simulink model "Aerosonde"  (R2025b)
settings: Solver=VariableStepAuto  StartTime=0.0  StopTime=100  RelTol=1e-3
values from neighbouring files (symbols this model uses):
  b = 2.8956    [init_params.m]    (also in init_params.mat)
  c = 0.18994    [init_params.m]    (also in init_params.mat)
  Cprop = 1.0    (= 1)    [init_params.m]    (also in init_params.mat)
  del_a = 0    [StatesAndInputs.m]
  del_e = 2*(pi/180)    (= 0.0349065850399)    [StatesAndInputs.m]
  del_r = 0    [StatesAndInputs.m]
  ForceCoefficients = [0.28 3.45 0 -0.36 0.03 0.3 0 0 0.0437 0 -0.98 0 ... (15 elements, 15x1)]    [init_params.mat]
  g = 9.80665    [init_params.m]    (also in init_params.mat)
  Ixx = 0.8244    [init_params.m]    (also in init_params.mat)
  Ixz = 0.1204    [init_params.m]    (also in init_params.mat)
  Iyy = 1.135    [init_params.m]    (also in init_params.mat)
  Izz = 1.759    [init_params.m]    (also in init_params.mat)
  k_motor = 80    [init_params.m]    (also in init_params.mat)
  k_omega = 0    [init_params.m]    (also in init_params.mat)
  k_Tp = 0    [init_params.m]    (also in init_params.mat)
  m = 13.5    [init_params.m]    (also in init_params.mat)
  MomentCoefficients = [0 -0.12 -0.26 0.14 0.08 0.105 -0.02338 -0.38 -3.6 -0.5 0 0.25 ... (16 elements, 16x1)]    [init_params.mat]
  p = 0    [StatesAndInputs.m]
  phi = 0    [StatesAndInputs.m]
  psi = 0    [StatesAndInputs.m]
  q = 0    [StatesAndInputs.m]
  r = 0    [StatesAndInputs.m]
  rho = 1.2682    [init_params.m]    (also in init_params.mat)
  S = 0.55    [init_params.m]    (also in init_params.mat)
  S_prop = 0.2027    [init_params.m]    (also in init_params.mat)
  theta = 3*(pi/180)    (= 0.0523598775598)    [StatesAndInputs.m]
  v = 0    [StatesAndInputs.m]
  w = 0    [StatesAndInputs.m]
  x = 0    [StatesAndInputs.m]
  y = 0    [StatesAndInputs.m]
  z = -50    [StatesAndInputs.m]
libraries: matrix_library x2, slpidlib x1
settings Model: Creator=deepa  LastModifiedBy=deepa
settings DataIOCC: ExternalInput=getinputstruct(op1)  InitialState=getstatestruct(op1)

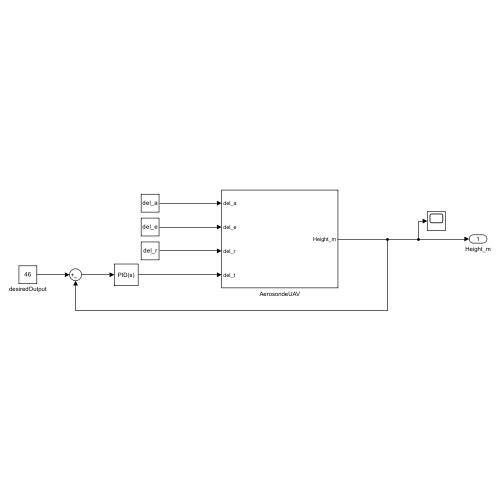
[thumbnail: Simulink's stored preview of the top-level diagram]
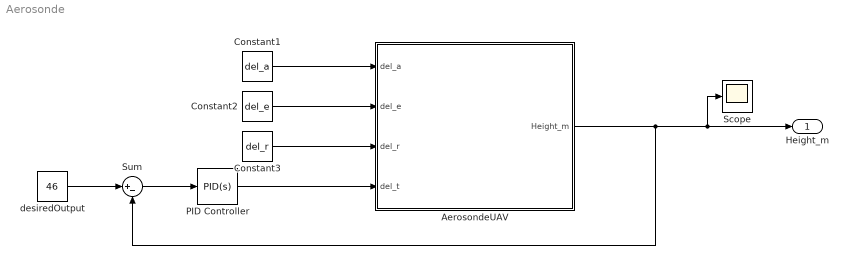
== system Aerosonde ==
  AerosondeUAV : Subsystem
  Constant1 : Constant  Value=del_a
  Constant2 : Constant  Value=del_e
  Constant3 : Constant  Value=del_r
  PID Controller : slpidlib/PID Controller  Controller=PID  Form=Parallel  TimeDomain=Continuous-time  UseExternalTs=off  SampleTime=-1  IntegratorMethod=Forward Euler  FilterMethod=Forward Euler  ControllerParametersSource=internal  P=1  I=1  UseKiTs=off  D=0  UseExternalDerivativeSource=off  N=100  UseFilter=on  TunerSelectOption=Transfer Function Based (PID Tuner App)  InitialConditionSource=internal  InitialConditionForIntegrator=0  InitialConditionForFilter=0  DifferentiatorICPrevScaledInput=0  ExternalReset=none  TrackingMode=off  Kt=1  LimitOutput=off  SatLimitsSource=internal  UpperSaturationLimit=inf  LowerSaturationLimit=-inf  LinearizeAsGain=on  AntiWindupMode=none  Kb=1  LimitIntegrator=off  UpperIntegratorSaturationLimit=inf  LowerIntegratorSaturationLimit=-inf  POutMin=[]  POutMax=[]  IOutMin=[]  IOutMax=[]  DOutMin=[]  DOutMax=[]  NOutMin=[]  NOutMax=[]  SumOutMin=[]  SumOutMax=[]  SaturationOutMin=[]  SaturationOutMax=[]  PParamMin=[]  PParamMax=[]  IParamMin=[]  IParamMax=[]  DParamMin=[]  DParamMax=[]  NParamMin=[]  NParamMax=[]  KbParamMin=[]  KbParamMax=[]  KtParamMin=[]  KtParamMax=[]  KbOutMin=[]  KbOutMax=[]  KtOutMin=[]  KtOutMax=[]  IntegratorOutMin=[]  IntegratorOutMax=[]  FilterOutMin=[]  FilterOutMax=[]  SumI1OutMin=[]  SumI1OutMax=[]  SumI2OutMin=[]  SumI2OutMax=[]  SumI3OutMin=[]  SumI3OutMax=[]  SumI4OutMin=[]  SumI4OutMax=[]  SumDOutMin=[]  SumDOutMax=[]  DifferentiatorOutMin=[]  DifferentiatorOutMax=[]  FilterDiffOutCoefMin=[]  FilterDiffOutCoefMax=[]  ReciprocalOutMin=[]  ReciprocalOutMax=[]  SumDenOutMin=[]  SumDenOutMax=[]  SumNumOutMin=[]  SumNumOutMax=[]  DivideOutMin=[]  DivideOutMax=[]  UdiffTsProdOutMin=[]  UdiffTsProdOutMax=[]  NTsProdOutMin=[]  NTsProdOutMax=[]  UintegralTsProdOutMin=[]  UintegralTsProdOutMax=[]  UngainTsProdOutMin=[]  UngainTsProdOutMax=[]  ClampingZeroOutDataTypeStr=Inherit: Inherit via back propagation  ClampingZeroOutMin=[]  ClampingZeroOutMax=[]  FilterDenConstantOutDataTypeStr=Inherit: Inherit via back propagation  FilterDenConstantOutMin=[]  FilterDenConstantOutMax=[]  PCopyOutDataTypeStr=Inherit: Inherit via back propagation  PCopyOutMin=[]  PCopyOutMax=[]  NCopyOutDataTypeStr=Inherit: Inherit via back propagation  NCopyOutMin=[]  NCopyOutMax=[]  IntegratorContinuousStateAttributes=''  IntegratorStateMustResolveToSignalObject=off  IntegratorRTWStateStorageClass=Auto  FilterContinuousStateAttributes=''  FilterStateMustResolveToSignalObject=off  FilterRTWStateStorageClass=Auto  ParallelPVariant=InternalParameters  IdealPVariant=Disabled  IVariant=InternalParameters  DVariant=InternalParameters  IntegratorVariant=Continuous  SatVariant=Disabled  AWVariant=Passthrough  PCopyVariant=Disabled  TRVariant=Disabled  FdbkBlocksVariant=Forward  IdealPFdbkVariant=Disabled  SatFdbkVariant=Disabled  DerivativeFilterVariant=ContFilter  NVariant=InternalParameters  NCopyVariant=Disabled  FilterICVariant=InternalICsFilter  IntegratorICVariant=InternalICs  ExternalResetVariant=Disabled  TRSumVariant=Passthrough  SumFdbkVariant=Disabled  SumVariant=Sum_PID  TsampFilterVariant=InternalTs  TsampNgainVariant=Passthrough  TsampIntegralVariant=Disabled_SignalSpec  ExternalSaturationOutDataTypeStr=Inherit: Same as second input  DerivativeSourceVariant=ErrorSignal  PreIntVariant=InternalPreInt
  Scope : Scope
      settings: ActiveDisplayYMinimum=-50.13744  ActiveDisplayYMaximum=-48.97284
  Sum : Sum  Inputs=|+-
  desiredOutput : Constant  Value=46
  Height_m : Outport
  wires:
  AerosondeUAV/1(Height_m) -> Sum/2, Scope/1, Height_m/1
  desiredOutput/1 -> Sum/1
  Constant1/1 -> AerosondeUAV/1(del_a)
  Constant2/1 -> AerosondeUAV/2(del_e)
  Constant3/1 -> AerosondeUAV/3(del_r)
  Sum/1 -> PID Controller/1
  PID Controller/1 -> AerosondeUAV/4(del_t)

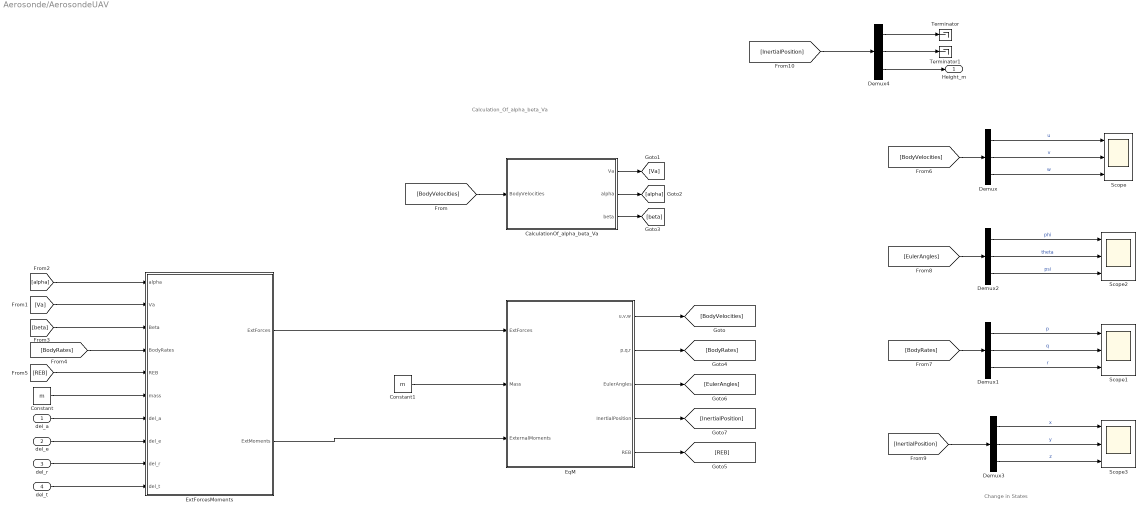
== system Aerosonde/AerosondeUAV ==
  note: Calculation_Of_alpha_beta_Va
  note: Change in States
  del_a : Inport
  del_e : Inport  Port=2
  del_r : Inport  Port=3
  del_t : Inport  Port=4
  CalculationOf_alpha_beta_Va : Subsystem
  Constant : Constant  Value=m
  Constant1 : Constant  Value=m
  Demux{,1..4} (5 alike) : Demux  Outputs=3
  EqM : Subsystem
  ExtForcesMoments : Subsystem
  Scope{,1..3} (4 alike) : Scope  NumInputPorts=3
      Scope settings: ActiveDisplayYMinimum=-68.28294  ActiveDisplayYMaximum=365.82044
      Scope1 settings: ActiveDisplayYMinimum=-3981.32854  ActiveDisplayYMaximum=442.36984
      Scope2 settings: ActiveDisplayYMinimum=-30055.42202  ActiveDisplayYMaximum=3339.54951  DataLoggingVariableName=ScopeData2
      Scope3 settings: ActiveDisplayYMinimum=-56.3817  ActiveDisplayYMaximum=7.22544  DataLoggingVariableName=ScopeData3
  Terminator : Terminator
  Terminator1 : Terminator
  Height_m : Outport
  wires:
  Constant/1 -> ExtForcesMoments/6(mass)
  EqM/3(EulerAngles) -> [EulerAngles]
  [beta] -> ExtForcesMoments/3(Beta)
  [InertialPosition] -> Demux3/1
  del_a/1 -> ExtForcesMoments/7(del_a)
  Demux4/2 -> Terminator1/1
  [REB] -> ExtForcesMoments/5(REB)
  EqM/2(p,q,r) -> [BodyRates]
  [Va] -> ExtForcesMoments/2(Va)
  Demux2/1 -> Scope2/1  "phi"
  Demux/2 -> Scope/2  "v"
  Demux3/2 -> Scope3/2  "y"
  Demux3/1 -> Scope3/1  "x"
  del_r/1 -> ExtForcesMoments/9(del_r)
  [BodyRates] -> ExtForcesMoments/4(BodyRates)
  [BodyRates] -> Demux1/1
  Constant1/1 -> EqM/2(Mass)
  CalculationOf_alpha_beta_Va/3(beta) -> [beta]
  [BodyVelocities] -> CalculationOf_alpha_beta_Va/1(BodyVelocities)
  [alpha] -> ExtForcesMoments/1(alpha)
  Demux3/3 -> Scope3/3  "z"
  Demux1/2 -> Scope1/2  "q"
  Demux/3 -> Scope/3  "w"
  Demux2/3 -> Scope2/3  "psi"
  Demux1/1 -> Scope1/1  "p"
  Demux/1 -> Scope/1  "u"
  EqM/4(InertialPosition) -> [InertialPosition]
  ExtForcesMoments/1(ExtForces) -> EqM/1(ExtForces)
  Demux2/2 -> Scope2/2  "theta"
  del_e/1 -> ExtForcesMoments/8(del_e)
  EqM/5(REB) -> [REB]
  EqM/1(u,v,w) -> [BodyVelocities]
  CalculationOf_alpha_beta_Va/1(Va) -> [Va]
  ExtForcesMoments/2(ExtMoments) -> EqM/3(ExternalMoments)
  [BodyVelocities] -> Demux/1
  CalculationOf_alpha_beta_Va/2(alpha) -> [alpha]
  [EulerAngles] -> Demux2/1
  Demux1/3 -> Scope1/3  "r"
  [InertialPosition] -> Demux4/1
  Demux4/1 -> Terminator/1
  Demux4/3 -> Height_m/1
  del_t/1 -> ExtForcesMoments/10(del_t)

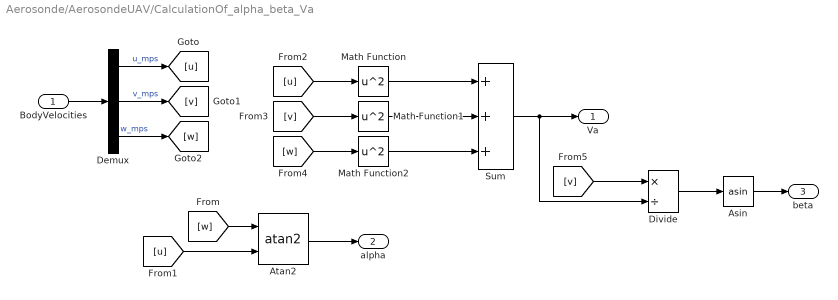
== system Aerosonde/AerosondeUAV/CalculationOf_alpha_beta_Va ==
  BodyVelocities : Inport
  Asin : Trigonometry  Operator=asin
  Atan2 : Trigonometry  Operator=atan2
  Demux : Demux  Outputs=3
  Divide : Product  Inputs=*/
  Math Function : Math  Operator=square
  Math Function1 : Math  Operator=square
  Math Function2 : Math  Operator=square
  Sum : Sum  Inputs=+++
  Va : Outport
  alpha : Outport  Port=2
  beta : Outport  Port=3
  wires:
  BodyVelocities/1 -> Demux/1
  Demux/1 -> [u]  "u_mps"
  Demux/2 -> [v]  "v_mps"
  Demux/3 -> [w]  "w_mps"
  [w] -> Atan2/1
  [u] -> Atan2/2
  Atan2/1 -> alpha/1
  [u] -> Math Function/1
  [v] -> Math Function1/1
  [w] -> Math Function2/1
  Math Function/1 -> Sum/1
  Math Function1/1 -> Sum/2
  Math Function2/1 -> Sum/3
  Sum/1 -> Divide/2, Va/1
  [v] -> Divide/1
  Divide/1 -> Asin/1
  Asin/1 -> beta/1

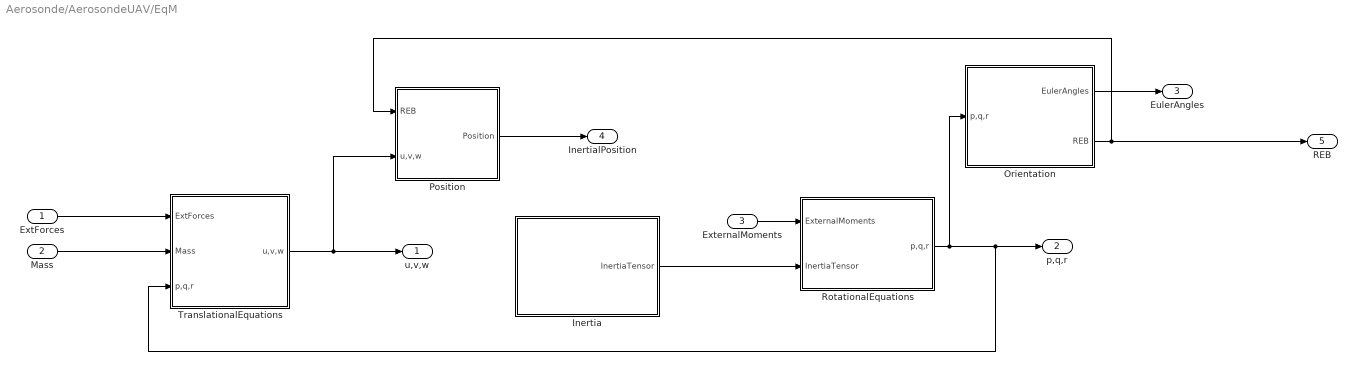
== system Aerosonde/AerosondeUAV/EqM ==
  ExtForces : Inport
  Mass : Inport  Port=2
  ExternalMoments : Inport  Port=3
  Inertia : Subsystem
  Orientation : Subsystem
  Position : Subsystem
  RotationalEquations : Subsystem
  TranslationalEquations : Subsystem
  u,v,w : Outport
  p,q,r : Outport  Port=2
  EulerAngles : Outport  Port=3
  InertialPosition : Outport  Port=4
  REB : Outport  Port=5
  wires:
  Orientation/2(REB) -> Position/1(REB), REB/1
  RotationalEquations/1(p,q,r) -> Orientation/1(p,q,r), p,q,r/1, TranslationalEquations/3(p,q,r)
  ExtForces/1 -> TranslationalEquations/1(ExtForces)
  Mass/1 -> TranslationalEquations/2(Mass)
  TranslationalEquations/1(u,v,w) -> u,v,w/1, Position/2(u,v,w)
  Orientation/1(EulerAngles) -> EulerAngles/1
  ExternalMoments/1 -> RotationalEquations/1(ExternalMoments)
  Inertia/1(InertiaTensor) -> RotationalEquations/2(InertiaTensor)
  Position/1(Position) -> InertialPosition/1

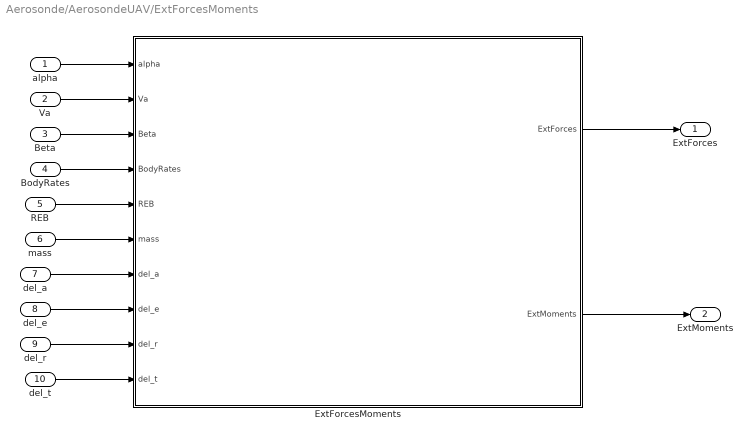
== system Aerosonde/AerosondeUAV/ExtForcesMoments ==
  alpha : Inport
  Va : Inport  Port=2
  Beta : Inport  Port=3
  BodyRates : Inport  Port=4
  REB : Inport  Port=5
  mass : Inport  Port=6
  del_a : Inport  Port=7
  del_e : Inport  Port=8
  del_r : Inport  Port=9
  del_t : Inport  Port=10
  ExtForcesMoments : Subsystem
  ExtForces : Outport
  ExtMoments : Outport  Port=2
  wires:
  alpha/1 -> ExtForcesMoments/1(alpha)
  Va/1 -> ExtForcesMoments/2(Va)
  Beta/1 -> ExtForcesMoments/3(Beta)
  BodyRates/1 -> ExtForcesMoments/4(BodyRates)
  REB/1 -> ExtForcesMoments/5(REB)
  mass/1 -> ExtForcesMoments/6(mass)
  del_a/1 -> ExtForcesMoments/7(del_a)
  del_e/1 -> ExtForcesMoments/8(del_e)
  del_r/1 -> ExtForcesMoments/9(del_r)
  del_t/1 -> ExtForcesMoments/10(del_t)
  ExtForcesMoments/1(ExtForces) -> ExtForces/1
  ExtForcesMoments/2(ExtMoments) -> ExtMoments/1

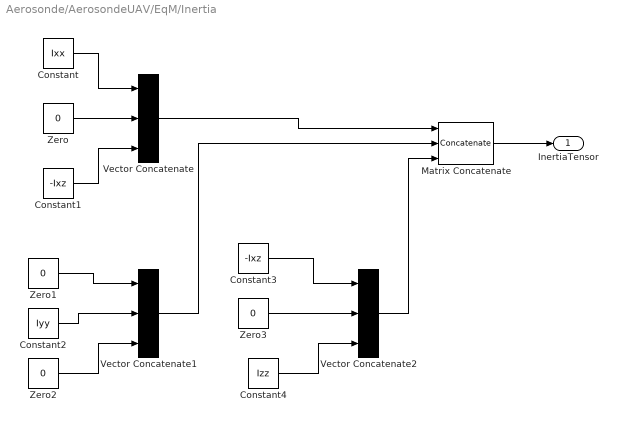
== system Aerosonde/AerosondeUAV/EqM/Inertia ==
  Constant : Constant  Value=Ixx
  Constant1 : Constant  Value=-Ixz
  Constant2 : Constant  Value=Iyy
  Constant3 : Constant  Value=-Ixz
  Constant4 : Constant  Value=Izz
  Matrix Concatenate : Concatenate  NumInputs=3  Mode=Multidimensional array  ConcatenateDimension=2
  Vector Concatenate : Concatenate  NumInputs=3  Mode=Multidimensional array
  Vector Concatenate1 : Concatenate  NumInputs=3  Mode=Multidimensional array
  Vector Concatenate2 : Concatenate  NumInputs=3  Mode=Multidimensional array
  Zero{,1..3} (4 alike) : Constant  Value=0  OutDataTypeStr=Inherit: Inherit via back propagation
  InertiaTensor : Outport
  wires:
  Zero2/1 -> Vector Concatenate1/3
  Constant3/1 -> Vector Concatenate2/1
  Constant2/1 -> Vector Concatenate1/2
  Zero/1 -> Vector Concatenate/2
  Constant1/1 -> Vector Concatenate/3
  Constant/1 -> Vector Concatenate/1
  Zero1/1 -> Vector Concatenate1/1
  Zero3/1 -> Vector Concatenate2/2
  Constant4/1 -> Vector Concatenate2/3
  Vector Concatenate/1 -> Matrix Concatenate/1
  Vector Concatenate1/1 -> Matrix Concatenate/2
  Vector Concatenate2/1 -> Matrix Concatenate/3
  Matrix Concatenate/1 -> InertiaTensor/1

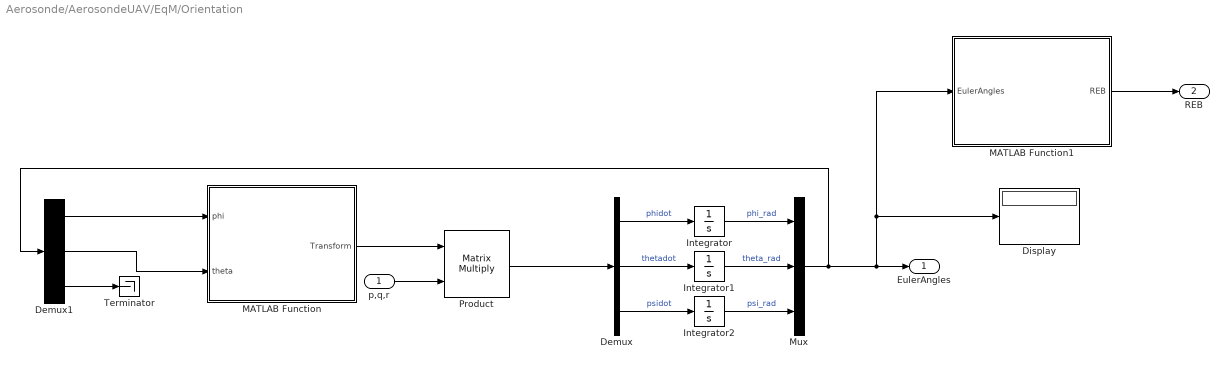
== system Aerosonde/AerosondeUAV/EqM/Orientation ==
  p,q,r : Inport
  Demux : Demux  Outputs=3
  Demux1 : Demux  Outputs=3
  Display : Display
  Integrator : Integrator  InitialCondition=phi  ContinuousStateAttributes='phi_rad'
  Integrator1 : Integrator  InitialCondition=theta  ContinuousStateAttributes='theta_rad'
  Integrator2 : Integrator  InitialCondition=psi  ContinuousStateAttributes='psi_rad'
  MATLAB Function : MATLAB Function  TreatAsAtomicUnit=on
  MATLAB Function1 : MATLAB Function  TreatAsAtomicUnit=on
  Mux : Mux  Inputs=3
  Product : Product  Multiplication=Matrix(*)
  Terminator : Terminator
  EulerAngles : Outport
  REB : Outport  Port=2
  wires:
  MATLAB Function/1(Transform) -> Product/1
  p,q,r/1 -> Product/2
  Product/1 -> Demux/1
  Demux/1 -> Integrator/1  "phidot"
  Demux/2 -> Integrator1/1  "thetadot"
  Demux/3 -> Integrator2/1  "psidot"
  Integrator/1 -> Mux/1  "phi_rad"
  Integrator1/1 -> Mux/2  "theta_rad"
  Integrator2/1 -> Mux/3  "psi_rad"
  Mux/1 -> Demux1/1, MATLAB Function1/1(EulerAngles), Display/1, EulerAngles/1
  MATLAB Function1/1(REB) -> REB/1
  Demux1/1 -> MATLAB Function/1(phi)
  Demux1/2 -> MATLAB Function/2(theta)
  Demux1/3 -> Terminator/1

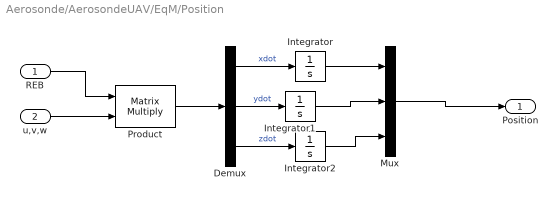
== system Aerosonde/AerosondeUAV/EqM/Position ==
  REB : Inport
  u,v,w : Inport  Port=2
  Demux : Demux  Outputs=3
  Integrator : Integrator  InitialCondition=x  ContinuousStateAttributes='x_m'
  Integrator1 : Integrator  InitialCondition=y  ContinuousStateAttributes='y_m'
  Integrator2 : Integrator  InitialCondition=z  ContinuousStateAttributes='z_m'
  Mux : Mux  Inputs=3
  Product : Product  Multiplication=Matrix(*)
  Position : Outport
  wires:
  REB/1 -> Product/1
  u,v,w/1 -> Product/2
  Product/1 -> Demux/1
  Demux/1 -> Integrator/1  "xdot"
  Demux/2 -> Integrator1/1  "ydot"
  Demux/3 -> Integrator2/1  "zdot"
  Integrator/1 -> Mux/1
  Integrator1/1 -> Mux/2
  Integrator2/1 -> Mux/3
  Mux/1 -> Position/1

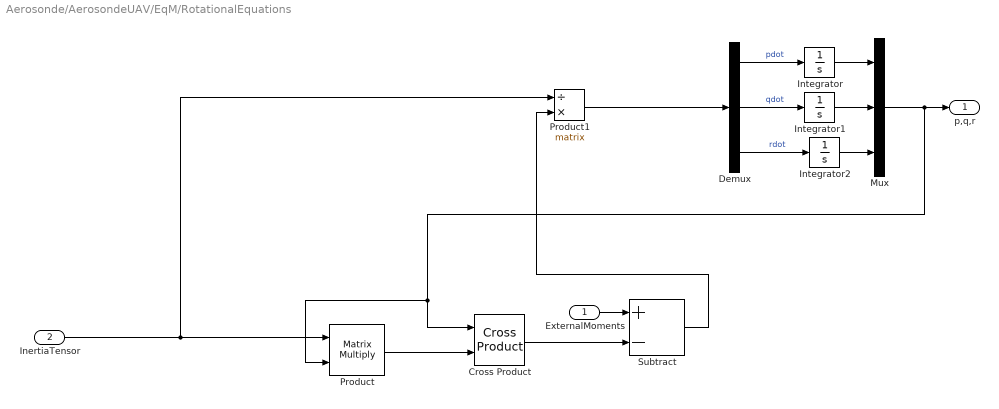
== system Aerosonde/AerosondeUAV/EqM/RotationalEquations ==
  ExternalMoments : Inport
  InertiaTensor : Inport  Port=2
  Cross Product : matrix_library/Cross Product
  Demux : Demux  Outputs=3
  Integrator : Integrator  InitialCondition=p  ContinuousStateAttributes='p_radps'
  Integrator1 : Integrator  InitialCondition=q  ContinuousStateAttributes='q_radps'
  Integrator2 : Integrator  InitialCondition=r  ContinuousStateAttributes='r_radps'
  Mux : Mux  Inputs=3
  Product : Product  Multiplication=Matrix(*)
  Product1 : Product  Inputs=/*  Multiplication=Matrix(*)
  Subtract : Sum  Inputs=+-
  p,q,r : Outport
  wires:
  Mux/1 -> Cross Product/1, Product/2, p,q,r/1
  InertiaTensor/1 -> Product1/1, Product/1
  ExternalMoments/1 -> Subtract/1
  Demux/1 -> Integrator/1  "pdot"
  Demux/2 -> Integrator1/1  "qdot"
  Demux/3 -> Integrator2/1  "rdot"
  Integrator2/1 -> Mux/3
  Integrator1/1 -> Mux/2
  Integrator/1 -> Mux/1
  Cross Product/1 -> Subtract/2
  Product/1 -> Cross Product/2
  Subtract/1 -> Product1/2
  Product1/1 -> Demux/1

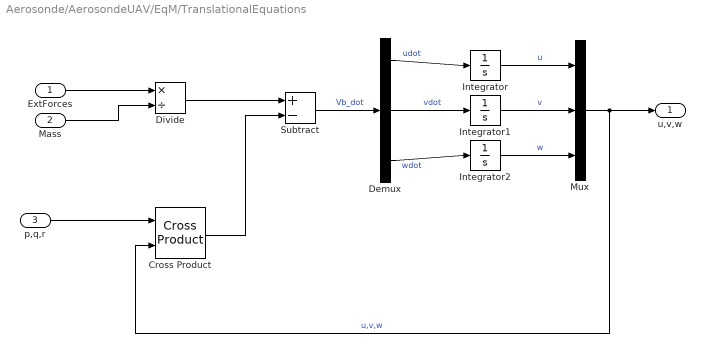
== system Aerosonde/AerosondeUAV/EqM/TranslationalEquations ==
  ExtForces : Inport
  Mass : Inport  Port=2
  p,q,r : Inport  Port=3
  Cross Product : matrix_library/Cross Product
  Demux : Demux  Outputs=3
  Divide : Product  Inputs=*/
  Integrator : Integrator  InitialCondition=u  ContinuousStateAttributes='u_mps'
  Integrator1 : Integrator  InitialCondition=v  ContinuousStateAttributes='v_mps'
  Integrator2 : Integrator  InitialCondition=w  ContinuousStateAttributes='w_mps'
  Mux : Mux  Inputs=3
  Subtract : Sum  Inputs=+-
  u,v,w : Outport
  wires:
  Integrator1/1 -> Mux/2  "v"
  Demux/2 -> Integrator1/1  "vdot"
  Mux/1 -> u,v,w/1, Cross Product/2  "u,v,w"
  ExtForces/1 -> Divide/1
  p,q,r/1 -> Cross Product/1
  Subtract/1 -> Demux/1  "Vb_dot"
  Integrator/1 -> Mux/1  "u"
  Demux/3 -> Integrator2/1  "wdot"
  Integrator2/1 -> Mux/3  "w"
  Mass/1 -> Divide/2
  Demux/1 -> Integrator/1  "udot"
  Cross Product/1 -> Subtract/2
  Divide/1 -> Subtract/1

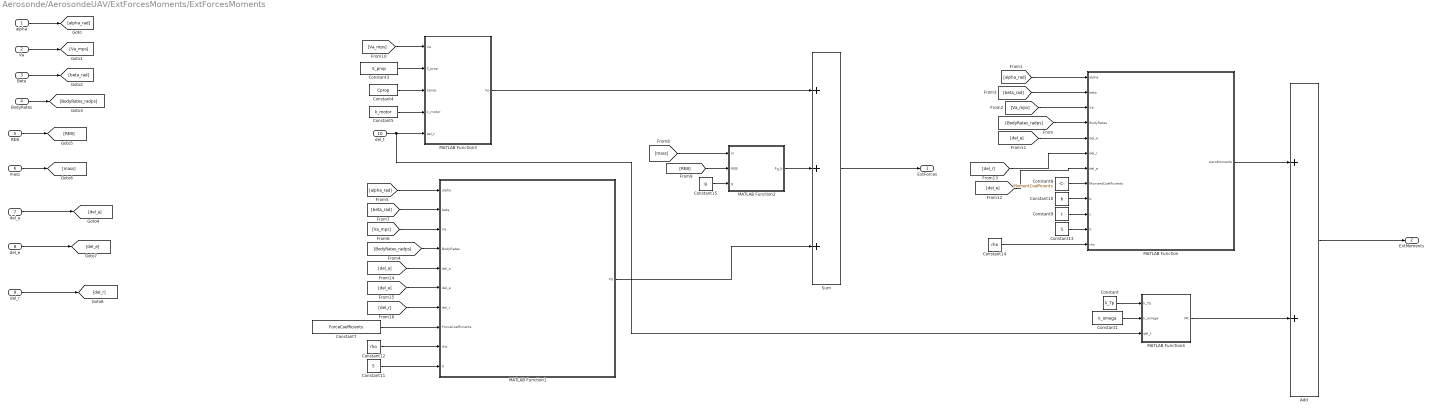
== system Aerosonde/AerosondeUAV/ExtForcesMoments/ExtForcesMoments ==
  alpha : Inport
  Va : Inport  Port=2
  Beta : Inport  Port=3
  BodyRates : Inport  Port=4
  REB : Inport  Port=5
  mass : Inport  Port=6
  del_a : Inport  Port=7
  del_e : Inport  Port=8
  del_r : Inport  Port=9
  del_t : Inport  Port=10
  Add : Sum
  Constant : Constant  Value=k_Tp
  Constant1 : Constant  Value=k_omega
  Constant10 : Constant  Value=b
  Constant11 : Constant  Value=S
  Constant12 : Constant  Value=rho
  Constant13 : Constant  Value=S
  Constant14 : Constant  Value=rho
  Constant15 : Constant  Value=g
  Constant3 : Constant  Value=S_prop
  Constant4 : Constant  Value=Cprop
  Constant5 : Constant  Value=k_motor
  Constant7 : Constant  Value=ForceCoefficients
  Constant8 : Constant  Value=MomentCoefficients
  Constant9 : Constant  Value=c
  MATLAB Function : MATLAB Function  TreatAsAtomicUnit=on
  MATLAB Function1 : MATLAB Function  TreatAsAtomicUnit=on
  MATLAB Function2 : MATLAB Function  TreatAsAtomicUnit=on
  MATLAB Function3 : MATLAB Function  TreatAsAtomicUnit=on
  MATLAB Function4 : MATLAB Function  TreatAsAtomicUnit=on
  Sum : Sum  Inputs=+++
  ExtForces : Outport
  ExtMoments : Outport  Port=2
  wires:
  Constant12/1 -> MATLAB Function1/9(rho)
  Constant3/1 -> MATLAB Function3/2(S_prop)
  MATLAB Function3/1(Fp) -> Sum/1
  Constant9/1 -> MATLAB Function/10(c)
  alpha/1 -> [alpha_rad]
  [Va_mps] -> MATLAB Function3/1(Va)
  [mass] -> MATLAB Function2/1(m)
  Sum/1 -> ExtForces/1
  [beta_rad] -> MATLAB Function1/2(beta)
  [alpha_rad] -> MATLAB Function/1(alpha)
  [del_e] -> MATLAB Function1/6(del_e)
  [del_e] -> MATLAB Function/7(del_e)
  Constant/1 -> MATLAB Function4/1(k_Tp)
  Beta/1 -> [beta_rad]
  Constant1/1 -> MATLAB Function4/2(k_omega)
  [del_r] -> MATLAB Function/6(del_r)
  Constant14/1 -> MATLAB Function/12(rho)
  mass/1 -> [mass]
  [del_a] -> MATLAB Function1/5(del_a)
  [BodyRates_radps] -> MATLAB Function1/4(BodyRates)
  Constant11/1 -> MATLAB Function1/10(S)
  MATLAB Function2/1(Fg_b) -> Sum/2
  Constant8/1 -> MATLAB Function/8(MomentCoefficients)
  del_e/1 -> [del_e]
  [alpha_rad] -> MATLAB Function1/1(alpha)
  Va/1 -> [Va_mps]
  MATLAB Function4/1(Mt) -> Add/2
  Constant15/1 -> MATLAB Function2/3(g)
  Constant7/1 -> MATLAB Function1/8(ForceCoefficients)
  [beta_rad] -> MATLAB Function/2(beta)
  BodyRates/1 -> [BodyRates_radps]
  [BodyRates_radps] -> MATLAB Function/4(BodyRates)
  [Va_mps] -> MATLAB Function1/3(Va)
  del_a/1 -> [del_a]
  [del_a] -> MATLAB Function/5(del_a)
  Constant4/1 -> MATLAB Function3/3(Cprop)
  Add/1 -> ExtMoments/1
  REB/1 -> [REB]
  MATLAB Function1/1(Fb) -> Sum/3
  Constant5/1 -> MATLAB Function3/4(k_motor)
  Constant10/1 -> MATLAB Function/9(b)
  [Va_mps] -> MATLAB Function/3(Va)
  [del_r] -> MATLAB Function1/7(del_r)
  MATLAB Function/1(AeroMoments) -> Add/1
  Constant13/1 -> MATLAB Function/11(S)
  del_t/1 -> MATLAB Function4/3(del_t), MATLAB Function3/5(del_t)
  [REB] -> MATLAB Function2/2(REB)
  del_r/1 -> [del_r]

== matlab function Aerosonde/AerosondeUAV/EqM/Orientation/MATLAB Function1 ==
  data: EulerAngles input; REB output
function REB = fcn(EulerAngles)

phi = EulerAngles(1);
theta = EulerAngles(2);
psi = EulerAngles(3);

REB = [cos(psi)*cos(theta)  cos(psi)*sin(theta)*sin(psi)-sin(psi)*cos(phi)  cos(psi)*sin(theta)*cos(phi)+sin(psi)*sin(phi);
       sin(psi)*cos(theta)  sin(psi)*sin(theta)*sin(phi)+cos(psi)*cos(phi)   sin(psi)*sin(theta)*cos(phi)-cos(psi)*sin(phi);
       -sin(theta)  cos(theta)*sin(phi) cos(theta)*cos(phi)];
end

== matlab function Aerosonde/AerosondeUAV/EqM/Orientation/MATLAB Function ==
  data: phi input; Transform output; theta input
function Transform = TransformMatrix(phi,theta)

   
    
    Transform = [1 tan(theta)*sin(phi) tan(theta)*cos(phi); ...
                 0 cos(phi) -sin(phi); ...
                 0 sec(theta)*sin(phi) sec(theta)*cos(phi)];


end

== matlab function Aerosonde/AerosondeUAV/ExtForcesMoments/ExtForcesMoments/MATLAB Function ==
  data: alpha input; AeroMoments output; beta input; Va input; BodyRates input; del_a input; del_r input; del_e input; MomentCoefficients input; b input; c input; S input; rho input
function AeroMoments = AerodynamicMoments(alpha, beta, Va, BodyRates, del_a, del_r, del_e,MomentCoefficients, b, c, S, rho)

p = BodyRates(1);
q = BodyRates(2);
r = BodyRates(3);

Cl0 = MomentCoefficients(1);
Cl_beta = MomentCoefficients(2);
Cl_p = MomentCoefficients(3);
Cl_r = MomentCoefficients(4);
Cl_del_a = MomentCoefficients(5);
Cl_del_r = MomentCoefficients(6);

Cm0 = MomentCoefficients(7);
Cm_alpha = MomentCoefficients(8); 
Cmq = MomentCoefficients(9);
Cm_del_e = MomentCoefficients(10);

Cn0 = MomentCoefficients(11);
Cn_beta = MomentCoefficients(12);
Cn_p = MomentCoefficients(13);
Cn_r = MomentCoefficients(14);
Cn_del_a = MomentCoefficients(15);
Cn_del_r = MomentCoefficients(16);

Cl = Cl0 + Cl_beta*beta + (Cl_p * b/(2*Va))*p + (Cl_r * b/(2*Va))*r + Cl_del_a*del_a + (Cl_del_r*del_r);

Cm = Cm0 + Cm_alpha*alpha + (Cmq * c/(2*Va))*q + Cm_del_e*del_e;

Cn = Cn0 + Cn_beta*beta + (Cn_p * b/(2*Va))*p + (Cn_r * b/(2*Va))*r + Cn_del_a*del_a + (Cn_del_r*del_r);

L = 0.5*rho*Va^2*S*b*Cl;

M = 0.5*rho*Va^2*S*c*Cm;

N = 0.5*rho*Va^2*S*b*Cn;


AeroMoments = [L;M;N];

end

== matlab function Aerosonde/AerosondeUAV/ExtForcesMoments/ExtForcesMoments/MATLAB Function1 ==
  data: alpha input; Fb output; beta input; Va input; BodyRates input; del_a input; del_e input; del_r input; ForceCoefficients input; rho input; S input
function Fb = AerodynamicForces(alpha, beta, Va, BodyRates, del_a, del_e, del_r, ForceCoefficients, rho, S)

CL0 = ForceCoefficients(1);
CL_alpha = ForceCoefficients(2);
CLq = ForceCoefficients(3);
CL_del_e = ForceCoefficients(4);
CD0 = ForceCoefficients(5);
CD_alpha = ForceCoefficients(6);
CDq = ForceCoefficients(7);
CD_del_e = ForceCoefficients(8);
CDp = ForceCoefficients(9);
CY0 = ForceCoefficients(10);
CY_beta = ForceCoefficients(11);
CYp = ForceCoefficients(12);
CY_r = ForceCoefficients(13);
CY_del_a = ForceCoefficients(14);
CY_del_r = ForceCoefficients(15);

p = BodyRates(1);
q = BodyRates(2);
r = BodyRates(3);


CL = CL0 + CL_alpha*alpha + CLq*q + CL_del_e*del_e;

CD = CD0 + CD_alpha*alpha^2 + CDq*q + CD_del_e*del_e + CDp*1;

CY = CY0 + CY_beta*beta + CYp*p + CY_r*r + CY_del_a*del_a + CY_del_r*del_r;

L = 0.5*rho*Va^2*S*CL;
Y = 0.5*rho*Va^2*S*CY;
D = 0.5*rho*Va^2*S*CD;

F_s = [-D;Y;-L];
C_bs = [cos(alpha) 0 -sin(alpha);
        0 1 0;
        sin(alpha) 0 cos(alpha)];

Fb = C_bs*F_s;

end

== matlab function Aerosonde/AerosondeUAV/ExtForcesMoments/ExtForcesMoments/MATLAB Function2 ==
  data: Fg_b output; m input; REB input; g input
function Fg_b = GravityForces(m,REB,g)


RBE = REB';

Fg_i = [0; 0; m*g];

Fg_b = RBE*Fg_i;

end

== matlab function Aerosonde/AerosondeUAV/ExtForcesMoments/ExtForcesMoments/MATLAB Function3 ==
  data: Va input; Fp output; S_prop input; Cprop input; k_motor input; del_t input
function Fp = PropulsiveForces(Va, S_prop,Cprop,k_motor, del_t)

Thrust = 0.5*S_prop*Cprop*((k_motor*del_t)^2 - Va^2);

Fp = [Thrust; 0; 0];

end

== matlab function Aerosonde/AerosondeUAV/ExtForcesMoments/ExtForcesMoments/MATLAB Function4 ==
  data: Mt output; k_Tp input; k_omega input; del_t input
function Mt = PropulsiveMoments(k_Tp,k_omega,del_t)

Mt = [-k_Tp*(k_omega*del_t)^2;
    0;
    0];

end
